simulink model "baskarModel"  (R2019a)
settings: Solver=VariableStepAuto  StartTime=0.0  StopTime=10.0  RelTol=1e-3
settings Model: Creator=darrahts  LastModifiedBy=darrahts

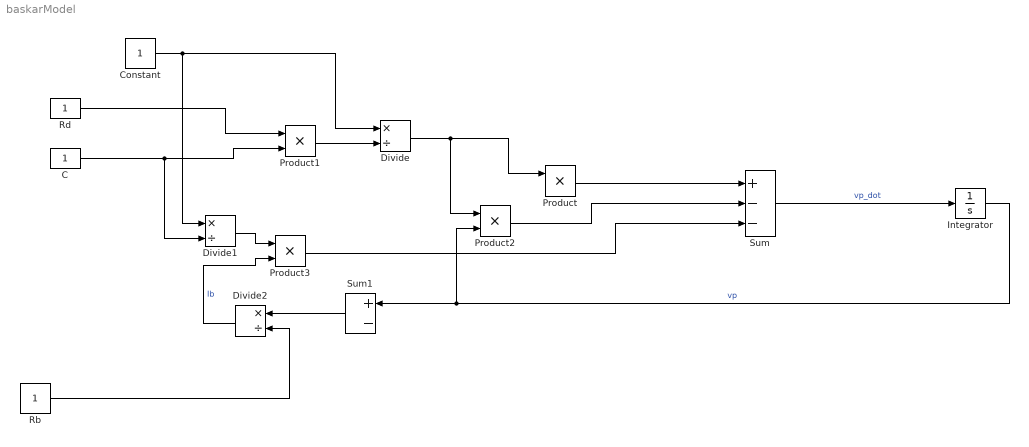
== system baskarModel ==
  C : Constant
  Constant : Constant
  Divide : Product  Inputs=*/
  Divide1 : Product  Inputs=*/
  Divide2 : Product  Inputs=*/
  Integrator : Integrator
  Product{,1..3} (4 alike) : Product
  Rb : Constant
  Rd : Constant
  Sum : Sum  Inputs=+--
  Sum1 : Sum  Inputs=+-
  wires:
  Integrator/1 -> Sum1/1, Product2/2  "vp"
  Sum/1 -> Integrator/1  "vp_dot"
  Divide/1 -> Product2/1, Product/1
  Product/1 -> Sum/1
  Constant/1 -> Divide1/1, Divide/1
  Product1/1 -> Divide/2
  Rd/1 -> Product1/1
  C/1 -> Divide1/2, Product1/2
  ? -> Product/2  "v0"
  Product2/1 -> Sum/2
  Product3/1 -> Sum/3
  Divide1/1 -> Product3/1
  Sum1/1 -> Divide2/1
  ? -> Sum1/2  "Vb"
  Rb/1 -> Divide2/2
  Divide2/1 -> Product3/2  "Ib"
